simulink model "Thirtybussys_final"  (R2023b)
settings: Solver=VariableStepAuto  StartTime=0.0  StopTime=0.7  RelTol=1e-3
libraries: eePowerMeasurement x60, spsFourierLib x60, spsThreePhaseSeriesRLCBranchLib x41, spsThreePhaseVIMeasurementLib x30, spsThreePhaseSeriesRLCLoadLib x21, spsThreePhaseSourceLib x6, spsThreePhaseTransformerTwoWindingsLib x6, spsThreePhaseFaultLib x2, spspowerguiLib x1
(part 1 of 3)
settings Model: Creator=sariy sh  LastModifiedBy=HP
settings SolverCC: AlgebraicLoopSolver=TrustRegion
settings DataIOCC: ReturnWorkspaceOutputs=off
settings DebuggingCC: UnconnectedInputMsg=warning  UnconnectedOutputMsg=warning  UnconnectedLineMsg=warning  ArithmeticOperatorsInVariantConditions=warning
settings ModelReferenceCC: EnableRefExpFcnMdlSchedulingChecks=on
settings SFSimCC: SimUseLocalCustomCode=off  CustomCodeUndefinedFunction=UseInterfaceOnly
settings RTWCC: RTWUseLocalCustomCode=off
settings CodeAppCC: StateflowObjectComments=on
settings SimscapeCC: SimscapeNormalizeSystem=off

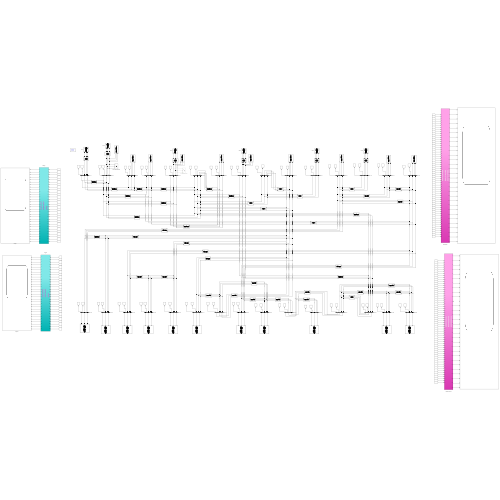
[thumbnail: Simulink's stored preview of the top-level diagram]
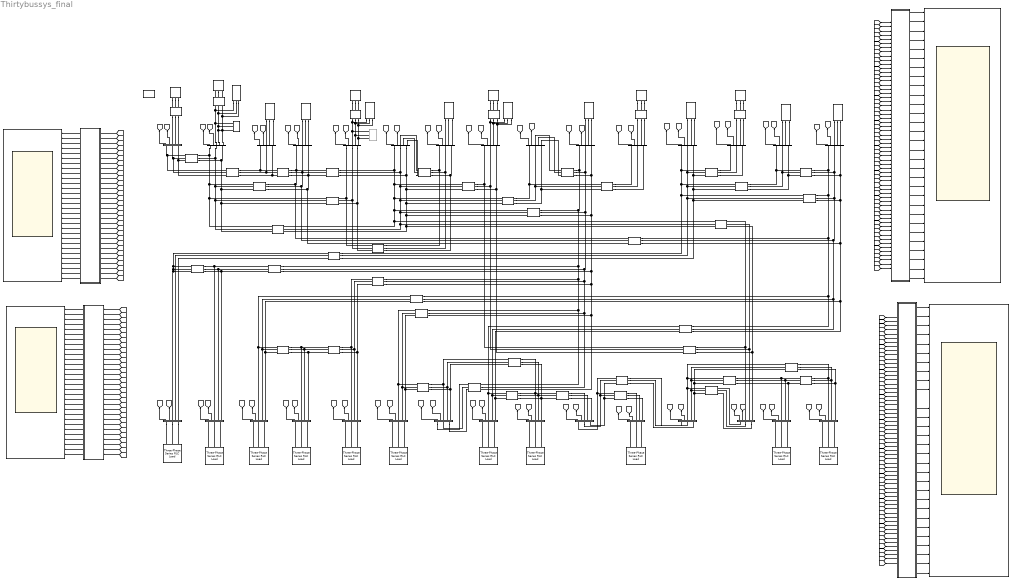
== system Thirtybussys_final ==
  " Reactive Power" : Subsystem
  " Real Power" : Subsystem
  Bus {1..30} (30 alike) : spsThreePhaseVIMeasurementLib/Three-Phase V-I Measurement  VoltageMeasurement=phase-to-ground  SetLabelV=off  LabelV=Vabc  Vpu=off  VpuLL=off  CurrentMeasurement=yes  SetLabelI=off  LabelI=Iabc  Ipu=off  Pbase=100e6  Vbase=500e3  OutputType=Complex  PhasorSimulation=off  PSBequivalent=0
  Current 1 : Subsystem
  Gen1 : spsThreePhaseSourceLib/Three-Phase Source  InternalConnection=Yg  VoltagePhases=off  Voltage=1.06  PhaseAngle=0  Voltage_phases=[25e3 25e3 25e3]/sqrt(3)  PhaseAngles_phases=[0 -120 +120]  Frequency=50  NonIdealSource=on  SpecifyImpedance=on  Resistance=0.8929  Inductance=16.58e-3  ShortCircuitLevel=100e6  BaseVoltage=1  XRratio=1  BusType=swing  Pref=10e3  Qref=0  Prefabc=[10e3, 10e3, 10e3]  Qrefabc=[0, 0, 0]  Qmin=-inf  Qmax=inf
  Gen2 : spsThreePhaseSourceLib/Three-Phase Source  InternalConnection=Yg  VoltagePhases=off  Voltage=1.045  PhaseAngle=0  Voltage_phases=[25e3 25e3 25e3]/sqrt(3)  PhaseAngles_phases=[0 -120 +120]  Frequency=50  NonIdealSource=on  SpecifyImpedance=on  Resistance=0.8929  Inductance=16.58e-3  ShortCircuitLevel=100e6  BaseVoltage=1  XRratio=1  BusType=PQ  Pref=0.4  Qref=0.5  Prefabc=[10e3, 10e3, 10e3]  Qrefabc=[0, 0, 0]  Qmin=-inf  Qmax=inf
  Gen3 : spsThreePhaseSourceLib/Three-Phase Source  InternalConnection=Yg  VoltagePhases=off  Voltage=1.010  PhaseAngle=0  Voltage_phases=[25e3 25e3 25e3]/sqrt(3)  PhaseAngles_phases=[0 -120 +120]  Frequency=50  NonIdealSource=on  SpecifyImpedance=on  Resistance=0.8929  Inductance=16.58e-3  ShortCircuitLevel=100e6  BaseVoltage=1  XRratio=1  BusType=PV  Pref=0.37  Qref=0  Prefabc=[10e3, 10e3, 10e3]  Qrefabc=[0, 0, 0]  Qmin=-0.15  Qmax=0.625
  Gen4 : spsThreePhaseSourceLib/Three-Phase Source  InternalConnection=Yg  VoltagePhases=off  Voltage=1.010  PhaseAngle=0  Voltage_phases=[25e3 25e3 25e3]/sqrt(3)  PhaseAngles_phases=[0 -120 +120]  Frequency=50  NonIdealSource=on  SpecifyImpedance=on  Resistance=0.8929  Inductance=16.58e-3  ShortCircuitLevel=100e6  BaseVoltage=1  XRratio=1  BusType=PV  Pref=0.373  Qref=0  Prefabc=[10e3, 10e3, 10e3]  Qrefabc=[0, 0, 0]  Qmin=-0.15  Qmax=0.50
  Gen5 : spsThreePhaseSourceLib/Three-Phase Source  InternalConnection=Yg  VoltagePhases=off  Voltage=1.082  PhaseAngle=0  Voltage_phases=[25e3 25e3 25e3]/sqrt(3)  PhaseAngles_phases=[0 -120 +120]  Frequency=50  NonIdealSource=on  SpecifyImpedance=on  Resistance=0.8929  Inductance=16.58e-3  ShortCircuitLevel=100e6  BaseVoltage=1  XRratio=1  BusType=PV  Pref=0.162  Qref=0  Prefabc=[10e3, 10e3, 10e3]  Qrefabc=[0, 0, 0]  Qmin=-0.10  Qmax=0.40
  Gen6 : spsThreePhaseSourceLib/Three-Phase Source  InternalConnection=Yg  VoltagePhases=off  Voltage=1.071  PhaseAngle=0  Voltage_phases=[25e3 25e3 25e3]/sqrt(3)  PhaseAngles_phases=[0 -120 +120]  Frequency=50  NonIdealSource=on  SpecifyImpedance=on  Resistance=0.8929  Inductance=16.58e-3  ShortCircuitLevel=100e6  BaseVoltage=1  XRratio=1  BusType=PV  Pref=0.106  Qref=0  Prefabc=[10e3, 10e3, 10e3]  Qrefabc=[0, 0, 0]  Qmin=-0.15  Qmax=0.45
  Reactive Power : Scope  NumInputPorts=30
  Real Power : Scope  NumInputPorts=30
  Scope1 : Scope  NumInputPorts=30
  Scope2 : Scope  NumInputPorts=30
  Three-Phase Series RLC Branch : spsThreePhaseSeriesRLCBranchLib/Three-Phase Series RLC Branch  LConnTagsString=A|B|C  RConnTagsString=A|B|C  BranchType=RLC  Resistance=0.0192  Inductance=0.0575/(2*pi*50)  Capacitance=1/0.0264/(2*pi*50)  Measurements=None
  Three-Phase Series RLC Branch1 : spsThreePhaseSeriesRLCBranchLib/Three-Phase Series RLC Branch  LConnTagsString=A|B|C  RConnTagsString=A|B|C  BranchType=RLC  Resistance=0.0452  Inductance=0.1652/(2*pi*50)  Capacitance=1/0.0204/(2*pi*50)  Measurements=None
  Three-Phase Series RLC Branch10 : spsThreePhaseSeriesRLCBranchLib/Three-Phase Series RLC Branch  LConnTagsString=A|B|C  RConnTagsString=A|B|C  BranchType=L  Resistance=0  Inductance=0.2080/(2*pi*50)  Capacitance=0  Measurements=None
  Three-Phase Series RLC Branch11 : spsThreePhaseSeriesRLCBranchLib/Three-Phase Series RLC Branch  LConnTagsString=A|B|C  RConnTagsString=A|B|C  BranchType=L  Resistance=1  Inductance=0.1100/(2*pi*50)  Capacitance=1e-6  Measurements=None
  Three-Phase Series RLC Branch12 : spsThreePhaseSeriesRLCBranchLib/Three-Phase Series RLC Branch  LConnTagsString=A|B|C  RConnTagsString=A|B|C  BranchType=L  Resistance=1  Inductance=0.5560/(2*pi*50)  Capacitance=1e-6  Measurements=None
  Three-Phase Series RLC Branch13 : spsThreePhaseSeriesRLCBranchLib/Three-Phase Series RLC Branch  LConnTagsString=A|B|C  RConnTagsString=A|B|C  BranchType=L  Resistance=1  Inductance=0.2080/(2*pi*50)  Capacitance=1e-6  Measurements=None
  Three-Phase Series RLC Branch14 : spsThreePhaseSeriesRLCBranchLib/Three-Phase Series RLC Branch  LConnTagsString=A|B|C  RConnTagsString=A|B|C  BranchType=L  Resistance=1  Inductance=0.1400/(2*pi*50)  Capacitance=1e-6  Measurements=None
  Three-Phase Series RLC Branch15 : spsThreePhaseSeriesRLCBranchLib/Three-Phase Series RLC Branch  LConnTagsString=A|B|C  RConnTagsString=A|B|C  BranchType=RL  Resistance=0.1231  Inductance=0.2559/(2*pi*50)  Capacitance=1e-6  Measurements=None
  Three-Phase Series RLC Branch16 : spsThreePhaseSeriesRLCBranchLib/Three-Phase Series RLC Branch  LConnTagsString=A|B|C  RConnTagsString=A|B|C  BranchType=RL  Resistance=0.2210  Inductance=0.1997/(2*pi*50)  Capacitance=1e-6  Measurements=None
  Three-Phase Series RLC Branch17 : spsThreePhaseSeriesRLCBranchLib/Three-Phase Series RLC Branch  LConnTagsString=A|B|C  RConnTagsString=A|B|C  BranchType=L  Resistance=1  Inductance=0.2560/(2*pi*50)  Capacitance=1e-6  Measurements=None
  Three-Phase Series RLC Branch18 : spsThreePhaseSeriesRLCBranchLib/Three-Phase Series RLC Branch  LConnTagsString=A|B|C  RConnTagsString=A|B|C  BranchType=RL  Resistance=0.0945  Inductance=0.1987/(2*pi*50)  Capacitance=1e-6  Measurements=None
  Three-Phase Series RLC Branch19 : spsThreePhaseSeriesRLCBranchLib/Three-Phase Series RLC Branch  LConnTagsString=A|B|C  RConnTagsString=A|B|C  BranchType=RLC  Resistance=0.0524  Inductance=0.1923/(2*pi*50)  Capacitance=1e-6  Measurements=None
  Three-Phase Series RLC Branch2 : spsThreePhaseSeriesRLCBranchLib/Three-Phase Series RLC Branch  LConnTagsString=A|B|C  RConnTagsString=A|B|C  BranchType=RLC  Resistance=0.0132  Inductance=0.0379/(2*pi*50)  Capacitance=1/0.0042/(2*pi*50)  Measurements=None
  Three-Phase Series RLC Branch20 : spsThreePhaseSeriesRLCBranchLib/Three-Phase Series RLC Branch  LConnTagsString=A|B|C  RConnTagsString=A|B|C  BranchType=RL  Resistance=0.0324  Inductance=0.0845/(2*pi*50)  Capacitance=1e-6  Measurements=None
  Three-Phase Series RLC Branch21 : spsThreePhaseSeriesRLCBranchLib/Three-Phase Series RLC Branch  LConnTagsString=A|B|C  RConnTagsString=A|B|C  BranchType=RL  Resistance=0.1063  Inductance=0.2185/(2*pi*50)  Capacitance=1e-6  Measurements=None
  Three-Phase Series RLC Branch22 : spsThreePhaseSeriesRLCBranchLib/Three-Phase Series RLC Branch  LConnTagsString=A|B|C  RConnTagsString=A|B|C  BranchType=RL  Resistance=0.0639  Inductance=0.1292/(2*pi*50)  Capacitance=1e-6  Measurements=None
  Three-Phase Series RLC Branch23 : spsThreePhaseSeriesRLCBranchLib/Three-Phase Series RLC Branch  LConnTagsString=A|B|C  RConnTagsString=A|B|C  BranchType=RL  Resistance=0.0340  Inductance=0.0680/(2*pi*50)  Capacitance=1e-6  Measurements=None
  Three-Phase Series RLC Branch24 : spsThreePhaseSeriesRLCBranchLib/Three-Phase Series RLC Branch  LConnTagsString=A|B|C  RConnTagsString=A|B|C  BranchType=RL  Resistance=0.0936  Inductance=0.2090/(2*pi*50)  Capacitance=1e-6  Measurements=None
  Three-Phase Series RLC Branch25 : spsThreePhaseSeriesRLCBranchLib/Three-Phase Series RLC Branch  LConnTagsString=A|B|C  RConnTagsString=A|B|C  BranchType=RL  Resistance=0.0348  Inductance=0.0749/(2*pi*50)  Capacitance=1e-6  Measurements=None
  Three-Phase Series RLC Branch26 : spsThreePhaseSeriesRLCBranchLib/Three-Phase Series RLC Branch  LConnTagsString=A|B|C  RConnTagsString=A|B|C  BranchType=RL  Resistance=0.0116  Inductance=0.0236/(2*pi*50)  Capacitance=1e-6  Measurements=None
  Three-Phase Series RLC Branch27 : spsThreePhaseSeriesRLCBranchLib/Three-Phase Series RLC Branch  LConnTagsString=A|B|C  RConnTagsString=A|B|C  BranchType=RL  Resistance=0.0727  Inductance=0.1499/(2*pi*50)  Capacitance=1e-6  Measurements=None
  Three-Phase Series RLC Branch28 : spsThreePhaseSeriesRLCBranchLib/Three-Phase Series RLC Branch  LConnTagsString=A|B|C  RConnTagsString=A|B|C  BranchType=RL  Resistance=0.1000  Inductance=0.2020/(2*pi*50)  Capacitance=1e-6  Measurements=None
  Three-Phase Series RLC Branch29 : spsThreePhaseSeriesRLCBranchLib/Three-Phase Series RLC Branch  LConnTagsString=A|B|C  RConnTagsString=A|B|C  BranchType=RL  Resistance=0.1150  Inductance=0.1790/(2*pi*50)  Capacitance=1e-6  Measurements=None
  Three-Phase Series RLC Branch3 : spsThreePhaseSeriesRLCBranchLib/Three-Phase Series RLC Branch  LConnTagsString=A|B|C  RConnTagsString=A|B|C  BranchType=RLC  Resistance=0.0570  Inductance=0.1737/(2*pi*50)  Capacitance=1/0.0184/(2*pi*50)  Measurements=None
  Three-Phase Series RLC Branch30 : spsThreePhaseSeriesRLCBranchLib/Three-Phase Series RLC Branch  LConnTagsString=A|B|C  RConnTagsString=A|B|C  BranchType=RL  Resistance=0.1320  Inductance=0.2700/(2*pi*50)  Capacitance=1e-6  Measurements=None
  Three-Phase Series RLC Branch31 : spsThreePhaseSeriesRLCBranchLib/Three-Phase Series RLC Branch  LConnTagsString=A|B|C  RConnTagsString=A|B|C  BranchType=RL  Resistance=0.1885  Inductance=0.3292/(2*pi*50)  Capacitance=1e-6  Measurements=None
  Three-Phase Series RLC Branch32 : spsThreePhaseSeriesRLCBranchLib/Three-Phase Series RLC Branch  LConnTagsString=A|B|C  RConnTagsString=A|B|C  BranchType=RL  Resistance=0.2544  Inductance=0.3800/(2*pi*50)  Capacitance=1e-6  Measurements=None
  Three-Phase Series RLC Branch33 : spsThreePhaseSeriesRLCBranchLib/Three-Phase Series RLC Branch  LConnTagsString=A|B|C  RConnTagsString=A|B|C  BranchType=RL  Resistance=0.1093  Inductance=0.2087/(2*pi*50)  Capacitance=1e-6  Measurements=None
  Three-Phase Series RLC Branch34 : spsThreePhaseSeriesRLCBranchLib/Three-Phase Series RLC Branch  LConnTagsString=A|B|C  RConnTagsString=A|B|C  BranchType=RL  Resistance=0.2198  Inductance=0.4153/(2*pi*50)  Capacitance=1e-6  Measurements=None
  Three-Phase Series RLC Branch35 : spsThreePhaseSeriesRLCBranchLib/Three-Phase Series RLC Branch  LConnTagsString=A|B|C  RConnTagsString=A|B|C  BranchType=RL  Resistance=0.3202  Inductance=0.6027/(2*pi*50)  Capacitance=1e-6  Measurements=None
  Three-Phase Series RLC Branch36 : spsThreePhaseSeriesRLCBranchLib/Three-Phase Series RLC Branch  LConnTagsString=A|B|C  RConnTagsString=A|B|C  BranchType=L  Resistance=1  Inductance=0.3960/(2*pi*50)  Capacitance=1e-6  Measurements=None
  Three-Phase Series RLC Branch37 : spsThreePhaseSeriesRLCBranchLib/Three-Phase Series RLC Branch  LConnTagsString=A|B|C  RConnTagsString=A|B|C  BranchType=RLC  Resistance=0.0169  Inductance=0.0599/(2*pi*50)  Capacitance=1/0.0065/(2*pi*50)  Measurements=None
  Three-Phase Series RLC Branch38 : spsThreePhaseSeriesRLCBranchLib/Three-Phase Series RLC Branch  LConnTagsString=A|B|C  RConnTagsString=A|B|C  BranchType=RLC  Resistance=0.0636  Inductance=0.2000/(2*pi*50)  Capacitance=1/0.0214/(2*pi*50)  Measurements=None
  Three-Phase Series RLC Branch39 : spsThreePhaseSeriesRLCBranchLib/Three-Phase Series RLC Branch  LConnTagsString=A|B|C  RConnTagsString=A|B|C  BranchType=RL  Resistance=0.0662  Inductance=0.1304/(2*pi*50)  Capacitance=1e-6  Measurements=None
  Three-Phase Series RLC Branch4 : spsThreePhaseSeriesRLCBranchLib/Three-Phase Series RLC Branch  LConnTagsString=A|B|C  RConnTagsString=A|B|C  BranchType=RLC  Resistance=0.0472  Inductance=0.1983/(2*pi*50)  Capacitance=1/0.0209/(2*pi*50)  Measurements=None
  Three-Phase Series RLC Branch40 : spsThreePhaseSeriesRLCBranchLib/Three-Phase Series RLC Branch  LConnTagsString=A|B|C  RConnTagsString=A|B|C  BranchType=RL  Resistance=0.2399  Inductance=0.4533/(2*pi*50)  Capacitance=1e-6  Measurements=None
  Three-Phase Series RLC Branch5 : spsThreePhaseSeriesRLCBranchLib/Three-Phase Series RLC Branch  LConnTagsString=A|B|C  RConnTagsString=A|B|C  BranchType=RLC  Resistance=0.0581  Inductance=0.1763/(2*pi*50)  Capacitance=1/0.0187/(2*pi*50)  Measurements=None
  Three-Phase Series RLC Branch6 : spsThreePhaseSeriesRLCBranchLib/Three-Phase Series RLC Branch  LConnTagsString=A|B|C  RConnTagsString=A|B|C  BranchType=RLC  Resistance=0.0119  Inductance=0.0414/(2*pi*50)  Capacitance=1/0.0045/(2*pi*50)  Measurements=None
  Three-Phase Series RLC Branch7 : spsThreePhaseSeriesRLCBranchLib/Three-Phase Series RLC Branch  LConnTagsString=A|B|C  RConnTagsString=A|B|C  BranchType=RLC  Resistance=0.0267  Inductance=0.0820/(2*pi*50)  Capacitance=1/0.0085/(2*pi*50)  Measurements=None
  Three-Phase Series RLC Branch8 : spsThreePhaseSeriesRLCBranchLib/Three-Phase Series RLC Branch  LConnTagsString=A|B|C  RConnTagsString=A|B|C  BranchType=RLC  Resistance=0.0460  Inductance=0.1160/(2*pi*50)  Capacitance=1/0.0102/(2*pi*50)  Measurements=None
  Three-Phase Series RLC Branch9 : spsThreePhaseSeriesRLCBranchLib/Three-Phase Series RLC Branch  LConnTagsString=A|B|C  RConnTagsString=A|B|C  BranchType=RLC  Resistance=0.0120  Inductance=0.0420/(2*pi*50)  Capacitance=1/0.0045/(2*pi*50)  Measurements=None
  Three-Phase Series RLC Load : spsThreePhaseSeriesRLCLoadLib/Three-Phase Series RLC Load  LConnTagsString=A|B|C  Configuration=Y (grounded)  NominalVoltage=1  Vabc=[1e3 1e3 1e3]  Vabcp=[1e3 1e3 1e3]  NominalFrequency=50  UnbalancedPower=off  ActivePower=0.217  InductivePower=0.127  CapacitivePower=0  Pabc=[10e3 9e3 11e3]  QLabc=[100 90 110]  QCabc=[100 90 110]  Pabcp=[10e3 9e3 11e3]  QLabcp=[100 90 110]  QCabcp=[100 90 110]  Measurements=None  LoadType=constant Z
  Three-Phase Series RLC Load1 : spsThreePhaseSeriesRLCLoadLib/Three-Phase Series RLC Load  LConnTagsString=A|B|C  Configuration=Y (grounded)  NominalVoltage=1  Vabc=[1e3 1e3 1e3]  Vabcp=[1e3 1e3 1e3]  NominalFrequency=50  UnbalancedPower=off  ActivePower=0.024  InductivePower=0.012  CapacitivePower=0  Pabc=[10e3 9e3 11e3]  QLabc=[100 90 110]  QCabc=[100 90 110]  Pabcp=[10e3 9e3 11e3]  QLabcp=[100 90 110]  QCabcp=[100 90 110]  Measurements=None  LoadType=constant Z
  Three-Phase Series RLC Load10 : spsThreePhaseSeriesRLCLoadLib/Three-Phase Series RLC Load  LConnTagsString=A|B|C  Configuration=Y (grounded)  NominalVoltage=1  Vabc=[1e3 1e3 1e3]  Vabcp=[1e3 1e3 1e3]  NominalFrequency=50  UnbalancedPower=off  ActivePower=0.062  InductivePower=0.016  CapacitivePower=0  Pabc=[10e3 9e3 11e3]  QLabc=[100 90 110]  QCabc=[100 90 110]  Pabcp=[10e3 9e3 11e3]  QLabcp=[100 90 110]  QCabcp=[100 90 110]  Measurements=None  LoadType=constant Z
  Three-Phase Series RLC Load11 : spsThreePhaseSeriesRLCLoadLib/Three-Phase Series RLC Load  LConnTagsString=A|B|C  Configuration=Y (grounded)  NominalVoltage=1  Vabc=[1e3 1e3 1e3]  Vabcp=[1e3 1e3 1e3]  NominalFrequency=50  UnbalancedPower=off  ActivePower=0.082  InductivePower=0.025  CapacitivePower=0  Pabc=[10e3 9e3 11e3]  QLabc=[100 90 110]  QCabc=[100 90 110]  Pabcp=[10e3 9e3 11e3]  QLabcp=[100 90 110]  QCabcp=[100 90 110]  Measurements=None  LoadType=constant Z
  Three-Phase Series RLC Load12 : spsThreePhaseSeriesRLCLoadLib/Three-Phase Series RLC Load  LConnTagsString=A|B|C  Configuration=Y (grounded)  NominalVoltage=1  Vabc=[1e3 1e3 1e3]  Vabcp=[1e3 1e3 1e3]  NominalFrequency=50  UnbalancedPower=off  ActivePower=0.3  InductivePower=0.3  CapacitivePower=0  Pabc=[10e3 9e3 11e3]  QLabc=[100 90 110]  QCabc=[100 90 110]  Pabcp=[10e3 9e3 11e3]  QLabcp=[100 90 110]  QCabcp=[100 90 110]  Measurements=None  LoadType=constant Z
  Three-Phase Series RLC Load13 : spsThreePhaseSeriesRLCLoadLib/Three-Phase Series RLC Load  LConnTagsString=A|B|C  Configuration=Y (grounded)  NominalVoltage=1  Vabc=[1e3 1e3 1e3]  Vabcp=[1e3 1e3 1e3]  NominalFrequency=50  UnbalancedPower=off  ActivePower=0.032  InductivePower=0.009  CapacitivePower=0  Pabc=[10e3 9e3 11e3]  QLabc=[100 90 110]  QCabc=[100 90 110]  Pabcp=[10e3 9e3 11e3]  QLabcp=[100 90 110]  QCabcp=[100 90 110]  Measurements=None  LoadType=constant Z
  Three-Phase Series RLC Load14 : spsThreePhaseSeriesRLCLoadLib/Three-Phase Series RLC Load  LConnTagsString=A|B|C  Configuration=Y (grounded)  NominalVoltage=1  Vabc=[1e3 1e3 1e3]  Vabcp=[1e3 1e3 1e3]  NominalFrequency=50  UnbalancedPower=off  ActivePower=0.095  InductivePower=0.034  CapacitivePower=0  Pabc=[10e3 9e3 11e3]  QLabc=[100 90 110]  QCabc=[100 90 110]  Pabcp=[10e3 9e3 11e3]  QLabcp=[100 90 110]  QCabcp=[100 90 110]  Measurements=None  LoadType=constant Z
  Three-Phase Series RLC Load15 : spsThreePhaseSeriesRLCLoadLib/Three-Phase Series RLC Load  LConnTagsString=A|B|C  Configuration=Y (grounded)  NominalVoltage=1  Vabc=[1e3 1e3 1e3]  Vabcp=[1e3 1e3 1e3]  NominalFrequency=50  UnbalancedPower=off  ActivePower=0.022  InductivePower=0.007  CapacitivePower=0  Pabc=[10e3 9e3 11e3]  QLabc=[100 90 110]  QCabc=[100 90 110]  Pabcp=[10e3 9e3 11e3]  QLabcp=[100 90 110]  QCabcp=[100 90 110]  Measurements=None  LoadType=constant Z
  Three-Phase Series RLC Load16 : spsThreePhaseSeriesRLCLoadLib/Three-Phase Series RLC Load  LConnTagsString=A|B|C  Configuration=Y (grounded)  NominalVoltage=1  Vabc=[1e3 1e3 1e3]  Vabcp=[1e3 1e3 1e3]  NominalFrequency=50  UnbalancedPower=off  ActivePower=0.175  InductivePower=0.112  CapacitivePower=0  Pabc=[10e3 9e3 11e3]  QLabc=[100 90 110]  QCabc=[100 90 110]  Pabcp=[10e3 9e3 11e3]  QLabcp=[100 90 110]  QCabcp=[100 90 110]  Measurements=None  LoadType=constant Z
  Three-Phase Series RLC Load17 : spsThreePhaseSeriesRLCLoadLib/Three-Phase Series RLC Load  LConnTagsString=A|B|C  Configuration=Y (grounded)  NominalVoltage=1  Vabc=[1e3 1e3 1e3]  Vabcp=[1e3 1e3 1e3]  NominalFrequency=50  UnbalancedPower=off  ActivePower=0.032  InductivePower=0.016  CapacitivePower=0  Pabc=[10e3 9e3 11e3]  QLabc=[100 90 110]  QCabc=[100 90 110]  Pabcp=[10e3 9e3 11e3]  QLabcp=[100 90 110]  QCabcp=[100 90 110]  Measurements=None  LoadType=constant Z
  Three-Phase Series RLC Load18 : spsThreePhaseSeriesRLCLoadLib/Three-Phase Series RLC Load  LConnTagsString=A|B|C  Configuration=Y (grounded)  NominalVoltage=1  Vabc=[1e3 1e3 1e3]  Vabcp=[1e3 1e3 1e3]  NominalFrequency=50  UnbalancedPower=off  ActivePower=0.087  InductivePower=0.067  CapacitivePower=0  Pabc=[10e3 9e3 11e3]  QLabc=[100 90 110]  QCabc=[100 90 110]  Pabcp=[10e3 9e3 11e3]  QLabcp=[100 90 110]  QCabcp=[100 90 110]  Measurements=None  LoadType=constant Z
  Three-Phase Series RLC Load19 : spsThreePhaseSeriesRLCLoadLib/Three-Phase Series RLC Load  LConnTagsString=A|B|C  Configuration=Y (grounded)  NominalVoltage=1  Vabc=[1e3 1e3 1e3]  Vabcp=[1e3 1e3 1e3]  NominalFrequency=50  UnbalancedPower=off  ActivePower=0.035  InductivePower=0.023  CapacitivePower=0  Pabc=[10e3 9e3 11e3]  QLabc=[100 90 110]  QCabc=[100 90 110]  Pabcp=[10e3 9e3 11e3]  QLabcp=[100 90 110]  QCabcp=[100 90 110]  Measurements=None  LoadType=constant Z
  Three-Phase Series RLC Load2 : spsThreePhaseSeriesRLCLoadLib/Three-Phase Series RLC Load  LConnTagsString=A|B|C  Configuration=Y (grounded)  NominalVoltage=1  Vabc=[1e3 1e3 1e3]  Vabcp=[1e3 1e3 1e3]  NominalFrequency=50  UnbalancedPower=off  ActivePower=0.076  InductivePower=0.016  CapacitivePower=0  Pabc=[10e3 9e3 11e3]  QLabc=[100 90 110]  QCabc=[100 90 110]  Pabcp=[10e3 9e3 11e3]  QLabcp=[100 90 110]  QCabcp=[100 90 110]  Measurements=None  LoadType=constant Z
  Three-Phase Series RLC Load21 : spsThreePhaseSeriesRLCLoadLib/Three-Phase Series RLC Load  LConnTagsString=A|B|C  Configuration=Y (grounded)  NominalVoltage=1  Vabc=[1e3 1e3 1e3]  Vabcp=[1e3 1e3 1e3]  NominalFrequency=50  UnbalancedPower=off  ActivePower=0.024  InductivePower=0.009  CapacitivePower=0  Pabc=[10e3 9e3 11e3]  QLabc=[100 90 110]  QCabc=[100 90 110]  Pabcp=[10e3 9e3 11e3]  QLabcp=[100 90 110]  QCabcp=[100 90 110]  Measurements=None  LoadType=constant Z
  Three-Phase Series RLC Load22 : spsThreePhaseSeriesRLCLoadLib/Three-Phase Series RLC Load  LConnTagsString=A|B|C  Configuration=Y (grounded)  NominalVoltage=1  Vabc=[1e3 1e3 1e3]  Vabcp=[1e3 1e3 1e3]  NominalFrequency=50  UnbalancedPower=off  ActivePower=0.106  InductivePower=0.019  CapacitivePower=0  Pabc=[10e3 9e3 11e3]  QLabc=[100 90 110]  QCabc=[100 90 110]  Pabcp=[10e3 9e3 11e3]  QLabcp=[100 90 110]  QCabcp=[100 90 110]  Measurements=None  LoadType=constant Z
  Three-Phase Series RLC Load3 : spsThreePhaseSeriesRLCLoadLib/Three-Phase Series RLC Load  LConnTagsString=A|B|C  Configuration=Y (grounded)  NominalVoltage=1  Vabc=[1e3 1e3 1e3]  Vabcp=[1e3 1e3 1e3]  NominalFrequency=50  UnbalancedPower=off  ActivePower=0.942  InductivePower=0.19  CapacitivePower=0  Pabc=[10e3 9e3 11e3]  QLabc=[100 90 110]  QCabc=[100 90 110]  Pabcp=[10e3 9e3 11e3]  QLabcp=[100 90 110]  QCabcp=[100 90 110]  Measurements=None  LoadType=constant Z
  Three-Phase Series RLC Load4 : spsThreePhaseSeriesRLCLoadLib/Three-Phase Series RLC Load  LConnTagsString=A|B|C  Configuration=Y (grounded)  NominalVoltage=1  Vabc=[1e3 1e3 1e3]  Vabcp=[1e3 1e3 1e3]  NominalFrequency=50  UnbalancedPower=off  ActivePower=0.09  InductivePower=0.058  CapacitivePower=0  Pabc=[10e3 9e3 11e3]  QLabc=[100 90 110]  QCabc=[100 90 110]  Pabcp=[10e3 9e3 11e3]  QLabcp=[100 90 110]  QCabcp=[100 90 110]  Measurements=None  LoadType=constant Z
  Three-Phase Series RLC Load5 : spsThreePhaseSeriesRLCLoadLib/Three-Phase Series RLC Load  LConnTagsString=A|B|C  Configuration=Y (grounded)  NominalVoltage=1  Vabc=[1e3 1e3 1e3]  Vabcp=[1e3 1e3 1e3]  NominalFrequency=50  UnbalancedPower=off  ActivePower=0.228  InductivePower=0.109  CapacitivePower=0  Pabc=[10e3 9e3 11e3]  QLabc=[100 90 110]  QCabc=[100 90 110]  Pabcp=[10e3 9e3 11e3]  QLabcp=[100 90 110]  QCabcp=[100 90 110]  Measurements=None  LoadType=constant Z
  Three-Phase Series RLC Load7 : spsThreePhaseSeriesRLCLoadLib/Three-Phase Series RLC Load  LConnTagsString=A|B|C  Configuration=Y (grounded)  NominalVoltage=1  Vabc=[1e3 1e3 1e3]  Vabcp=[1e3 1e3 1e3]  NominalFrequency=50  UnbalancedPower=off  ActivePower=0.058  InductivePower=0.02  CapacitivePower=0  Pabc=[10e3 9e3 11e3]  QLabc=[100 90 110]  QCabc=[100 90 110]  Pabcp=[10e3 9e3 11e3]  QLabcp=[100 90 110]  QCabcp=[100 90 110]  Measurements=None  LoadType=constant Z
  Three-Phase Series RLC Load8 : spsThreePhaseSeriesRLCLoadLib/Three-Phase Series RLC Load  LConnTagsString=A|B|C  Configuration=Y (grounded)  NominalVoltage=1  Vabc=[1e3 1e3 1e3]  Vabcp=[1e3 1e3 1e3]  NominalFrequency=50  UnbalancedPower=off  ActivePower=0.09  InductivePower=0.058  CapacitivePower=0  Pabc=[10e3 9e3 11e3]  QLabc=[100 90 110]  QCabc=[100 90 110]  Pabcp=[10e3 9e3 11e3]  QLabcp=[100 90 110]  QCabcp=[100 90 110]  Measurements=None  LoadType=constant Z
  Three-Phase Series RLC Load9 : spsThreePhaseSeriesRLCLoadLib/Three-Phase Series RLC Load  LConnTagsString=A|B|C  Configuration=Y (grounded)  NominalVoltage=1  Vabc=[1e3 1e3 1e3]  Vabcp=[1e3 1e3 1e3]  NominalFrequency=50  UnbalancedPower=off  ActivePower=0.112  InductivePower=0.075  CapacitivePower=0  Pabc=[10e3 9e3 11e3]  QLabc=[100 90 110]  QCabc=[100 90 110]  Pabcp=[10e3 9e3 11e3]  QLabcp=[100 90 110]  QCabcp=[100 90 110]  Measurements=None  LoadType=constant Z
  Three-Phase Transformer (Two Windings) : spsThreePhaseTransformerTwoWindingsLib/Three-Phase Transformer (Two Windings)  Winding1Connection=Yg  Winding2Connection=Yg  CoreType=Three single-phase transformers  SetSaturation=off  Hysteresis=off  DataFile='hysteresis'  SetInitialFlux=off  Measurements=None  UNITS=pu  NominalPower=[ 1 , 50 ]  Winding1=[1.06 , 0.002 , 0.08 ]  Winding2=[ 1.06 , 0.002 , 0.08 ]  Rm=500  Lm=500  L0=0.5  Saturation=[ 0,0 ; 0.0024,1.2 ; 1.0,1.52 ]  InitialFluxes=[ 0.8 , -0.8 , 0.7 ]  BreakLoop=off  DiscreteSolver=Trapezoidal iterative  DataType=off  TransfoNumber=1
  Three-Phase Transformer (Two Windings)1 : spsThreePhaseTransformerTwoWindingsLib/Three-Phase Transformer (Two Windings)  Winding1Connection=Yg  Winding2Connection=Yg  CoreType=Three single-phase transformers  SetSaturation=off  Hysteresis=off  DataFile='hysteresis'  SetInitialFlux=off  Measurements=None  UNITS=pu  NominalPower=[1 , 50 ]  Winding1=[ 1.045 , 0.002 , 0.08 ]  Winding2=[ 1.045 , 0.002 , 0.08 ]  Rm=500  Lm=500  L0=0.5  Saturation=[ 0,0 ; 0.0024,1.2 ; 1.0,1.52 ]  InitialFluxes=[ 0.8 , -0.8 , 0.7 ]  BreakLoop=off  DiscreteSolver=Trapezoidal iterative  DataType=off  TransfoNumber=1
  Three-Phase Transformer (Two Windings)2 : spsThreePhaseTransformerTwoWindingsLib/Three-Phase Transformer (Two Windings)  Winding1Connection=Yg  Winding2Connection=Yg  CoreType=Three single-phase transformers  SetSaturation=off  Hysteresis=off  DataFile='hysteresis'  SetInitialFlux=off  Measurements=None  UNITS=pu  NominalPower=[ 1 , 50 ]  Winding1=[ 1.010 , 0.002 , 0.08 ]  Winding2=[ 1.010 , 0.002 , 0.08 ]  Rm=500  Lm=500  L0=0.5  Saturation=[ 0,0 ; 0.0024,1.2 ; 1.0,1.52 ]  InitialFluxes=[ 0.8 , -0.8 , 0.7 ]  BreakLoop=off  DiscreteSolver=Trapezoidal iterative  DataType=off  TransfoNumber=1
  Three-Phase Transformer (Two Windings)3 : spsThreePhaseTransformerTwoWindingsLib/Three-Phase Transformer (Two Windings)  Winding1Connection=Yg  Winding2Connection=Yg  CoreType=Three single-phase transformers  SetSaturation=off  Hysteresis=off  DataFile='hysteresis'  SetInitialFlux=off  Measurements=None  UNITS=pu  NominalPower=[ 250e6 , 60 ]  Winding1=[ 735e3 , 0.002 , 0.08 ]  Winding2=[ 315e3 , 0.002 , 0.08 ]  Rm=500  Lm=500  L0=0.5  Saturation=[ 0,0 ; 0.0024,1.2 ; 1.0,1.52 ]  InitialFluxes=[ 0.8 , -0.8 , 0.7 ]  BreakLoop=off  DiscreteSolver=Trapezoidal iterative  DataType=off  TransfoNumber=1
  Three-Phase Transformer (Two Windings)4 : spsThreePhaseTransformerTwoWindingsLib/Three-Phase Transformer (Two Windings)  Winding1Connection=Yg  Winding2Connection=Yg  CoreType=Three single-phase transformers  SetSaturation=off  Hysteresis=off  DataFile='hysteresis'  SetInitialFlux=off  Measurements=None  UNITS=pu  NominalPower=[ 1 , 50 ]  Winding1=[ 1.082 , 0.002 , 0.08 ]  Winding2=[ 1.082 , 0.002 , 0.08 ]  Rm=500  Lm=500  L0=0.5  Saturation=[ 0,0 ; 0.0024,1.2 ; 1.0,1.52 ]  InitialFluxes=[ 0.8 , -0.8 , 0.7 ]  BreakLoop=off  DiscreteSolver=Trapezoidal iterative  DataType=off  TransfoNumber=1
  Three-Phase Transformer (Two Windings)5 : spsThreePhaseTransformerTwoWindingsLib/Three-Phase Transformer (Two Windings)  Winding1Connection=Yg  Winding2Connection=Yg  CoreType=Three single-phase transformers  SetSaturation=off  Hysteresis=off  DataFile='hysteresis'  SetInitialFlux=off  Measurements=None  UNITS=pu  NominalPower=[ 1 , 50 ]  Winding1=[ 1.071 , 0.002 , 0.08 ]  Winding2=[ 1.071 , 0.002 , 0.08 ]  Rm=500  Lm=500  L0=0.5  Saturation=[ 0,0 ; 0.0024,1.2 ; 1.0,1.52 ]  InitialFluxes=[ 0.8 , -0.8 , 0.7 ]  BreakLoop=off  DiscreteSolver=Trapezoidal iterative  DataType=off  TransfoNumber=1
  Three-Phase Fault1 : spsThreePhaseFaultLib/Three-Phase Fault  Commented=on  InitialStates=0  FaultA=on  FaultB=on  FaultC=on  GroundFault=on  SwitchTimes="[0.4  0.5]"  External=off  SwitchStatus=NaN  FaultResistance=0.001  GroundResistance=0.01  SnubberResistance=1e6  SnubberCapacitance=inf  Measurements=None
  Three-Phase Fault2 : spsThreePhaseFaultLib/Three-Phase Fault  InitialStates=0  FaultA=on  FaultB=on  FaultC=on  GroundFault=on  SwitchTimes="[0.4  0.5]"  External=off  SwitchStatus=NaN  FaultResistance=0.01  GroundResistance=0.01  SnubberResistance=1e6  SnubberCapacitance=inf  Measurements=None
  "Voltage " : Subsystem
  powergui : spspowerguiLib/powergui  Priority=1  SimulationMode=Discrete  SampleTime=50e-6  frequency=60  Iterations=50  frequencyindice=50  Pbase=100e6  ErrMax=1e-4  UnitsV=kV  UnitsW=MW  buscounter=0  FunctionMessages=off  echomessages=off  EnableUseOfTLC=off  CurrentSourceSwitches=off  DisableSnubberDevices=off  DisableRonSwitches=off  DisableVfSwitches=off  DisplayEquations=off  AutomaticDiscreteSolvers=off  SolverType=Tustin/Backward Euler (TBE)  Interpol=off  ExternalGateDelay=off  methode=off  Ts=100  x0status=blocks  SPID=off  SwTol=0  HookPort=off  NonlinearTolerance=1e-4  nMaxIteration=100  ContinueOnMaxIteration=off  RestoreLinks=warning  ResistiveCurrentMeasurement=off  Frange=[0:2:500]  Ylog=off  Xlog=on  ShowGrid=off  save=off  variable=ZData  structure=0  ZoomFFT=off  StartTime=0.0  cycles=1  DisplayStyle=1  fundamental=60  FreqAxis=off  MaxFrequency=1000  frequencyindicesteady=1  RmsSteady=1  display=off
  wires:
  Bus 4/1 -> [V4]
  Bus 4/2 -> [I4]
  Bus 5/1 -> [V5]
  Bus 5/2 -> [I5]
  Bus 6/1 -> [V6]
  Bus 6/2 -> [I6]
  Bus 12/1 -> [V12]
  Bus 12/2 -> [I12]
  Bus 13/1 -> [V13]
  Bus 13/2 -> [I13]
  Bus 14/1 -> [V14]
  Bus 14/2 -> [I14]
  Bus 15/1 -> [V15]
  Bus 15/2 -> [I15]
  Bus 16/1 -> [V16]
  Bus 16/2 -> [I16]
  Bus 17/1 -> [V17]
  Bus 17/2 -> [I17]
  Bus 18/1 -> [V18]
  Bus 18/2 -> [I18]
  Bus 19/1 -> [V19]
  Bus 19/2 -> [I19]
  Bus 20/1 -> [V20]
  Bus 20/2 -> [I20]
  Bus 21/1 -> [V21]
  Bus 21/2 -> [I21]
  Bus 22/1 -> [V22]
  Bus 22/2 -> [I22]
  Bus 23/1 -> [V23]
  Bus 23/2 -> [I23]
  Bus 24/1 -> [V24]
  Bus 24/2 -> [I24]
  Bus 25/1 -> [V25]
  Bus 25/2 -> [I25]
  Bus 26/1 -> [V26]
  Bus 26/2 -> [I26]
  Bus 27/1 -> [V27]
  Bus 27/2 -> [I27]
  Bus 28/1 -> [V28]
  Bus 28/2 -> [I28]
  Bus 29/1 -> [V29]
  Bus 29/2 -> [I29]
  Bus 30/1 -> [V30]
  Bus 30/2 -> [I30]
  Bus 2/2 -> [I2]
  Bus 3/2 -> [I3]
  Bus 3/1 -> [V3]
  Bus 1/2 -> [I1]
  Bus 1/1 -> [V1]
  Bus 2/1 -> [V2]
  Bus 7/1 -> [V7]
  Bus 8/1 -> [V8]
  Bus 9/1 -> [V9]
  Bus 10/1 -> [V10]
  Bus 7/2 -> [I7]
  Bus 8/2 -> [I8]
  Bus 9/2 -> [I9]
  Bus 10/2 -> [I10]
  Bus 11/1 -> [V11]
  Bus 11/2 -> [I11]
  [I7] -> Current 1/7(In7)
  [I26] -> Current 1/26(In26)
  [V18] -> "Voltage "/18(In18)
  [V14] -> "Voltage "/14(In14)
  "Voltage "/14(Out14) -> Scope1/14
  "Voltage "/24(Out24) -> Scope1/24
  "Voltage "/10(Out10) -> Scope1/10
  "Voltage "/17(Out17) -> Scope1/17
  "Voltage "/29(Out29) -> Scope1/29
  "Voltage "/16(Out16) -> Scope1/16
  [V11] -> "Voltage "/11(In11)
  "Voltage "/5(Out5) -> Scope1/5
  "Voltage "/20(Out20) -> Scope1/20
  [V3] -> "Voltage "/3(In3)
  [V10] -> "Voltage "/10(In10)
  "Voltage "/21(Out21) -> Scope1/21
  "Voltage "/26(Out26) -> Scope1/26
  [V21] -> "Voltage "/21(In21)
  [V9] -> "Voltage "/9(In9)
  "Voltage "/9(Out9) -> Scope1/9
  "Voltage "/7(Out7) -> Scope1/7
  "Voltage "/23(Out23) -> Scope1/23
  "Voltage "/30(Out30) -> Scope1/30
  "Voltage "/6(Out6) -> Scope1/6
  "Voltage "/22(Out22) -> Scope1/22
  "Voltage "/28(Out28) -> Scope1/28
  [V19] -> "Voltage "/19(In19)
  "Voltage "/8(Out8) -> Scope1/8
  [V1] -> "Voltage "/1(In1)
  [V6] -> "Voltage "/6(In6)
  [V26] -> "Voltage "/26(In26)
  [V20] -> "Voltage "/20(In20)
  [V27] -> "Voltage "/27(In27)
  "Voltage "/15(Out15) -> Scope1/15
  [V25] -> "Voltage "/25(In25)
  [V28] -> "Voltage "/28(In28)
  "Voltage "/13(Out13) -> Scope1/13
  [V4] -> "Voltage "/4(In4)
  [V5] -> "Voltage "/5(In5)
  [V29] -> "Voltage "/29(In29)
  [V7] -> "Voltage "/7(In7)
  [V8] -> "Voltage "/8(In8)
  [V16] -> "Voltage "/16(In16)
  "Voltage "/19(Out19) -> Scope1/19
  [V30] -> "Voltage "/30(In30)
  "Voltage "/12(Out12) -> Scope1/12
  [V13] -> "Voltage "/13(In13)
  "Voltage "/11(Out11) -> Scope1/11
  "Voltage "/3(Out3) -> Scope1/3
  [V2] -> "Voltage "/2(In2)
  "Voltage "/27(Out27) -> Scope1/27
  "Voltage "/2(Out2) -> Scope1/2
  [V15] -> "Voltage "/15(In15)
  "Voltage "/1(Out1) -> Scope1/1
  "Voltage "/18(Out18) -> Scope1/18
  [V24] -> "Voltage "/24(In24)
  [V22] -> "Voltage "/22(In22)
  [I9] -> Current 1/9(In9)
  [I8] -> Current 1/8(In8)
  [I13] -> Current 1/13(In13)
  [I3] -> Current 1/3(In3)
  [I14] -> Current 1/14(In14)
  [I4] -> Current 1/4(In4)
  [I10] -> Current 1/10(In10)
  Current 1/22(Out22) -> Scope2/22
  Current 1/7(Out7) -> Scope2/7
  Current 1/9(Out9) -> Scope2/9
  Current 1/14(Out14) -> Scope2/14
  Current 1/18(Out18) -> Scope2/18
  [I29] -> Current 1/29(In29)
  "Voltage "/4(Out4) -> Scope1/4
  Current 1/25(Out25) -> Scope2/25
  Current 1/4(Out4) -> Scope2/4
  Current 1/29(Out29) -> Scope2/29
  "Voltage "/25(Out25) -> Scope1/25
  [I15] -> Current 1/15(In15)
  Current 1/21(Out21) -> Scope2/21
  [I6] -> Current 1/6(In6)
  [I30] -> Current 1/30(In30)
  Current 1/15(Out15) -> Scope2/15
  Current 1/19(Out19) -> Scope2/19
  Current 1/13(Out13) -> Scope2/13
  [V12] -> "Voltage "/12(In12)
  Current 1/20(Out20) -> Scope2/20
  Current 1/30(Out30) -> Scope2/30
  [I18] -> Current 1/18(In18)
  Current 1/3(Out3) -> Scope2/3
  Current 1/6(Out6) -> Scope2/6
  Current 1/26(Out26) -> Scope2/26
  Current 1/23(Out23) -> Scope2/23
  Current 1/16(Out16) -> Scope2/16
  Current 1/24(Out24) -> Scope2/24
  Current 1/10(Out10) -> Scope2/10
  [I5] -> Current 1/5(In5)
  [I28] -> Current 1/28(In28)
  Current 1/5(Out5) -> Scope2/5
  Current 1/28(Out28) -> Scope2/28
  Current 1/1(Out1) -> Scope2/1
  Current 1/11(Out11) -> Scope2/11
  [I25] -> Current 1/25(In25)
  [I17] -> Current 1/17(In17)
  [I27] -> Current 1/27(In27)
  Current 1/2(Out2) -> Scope2/2
  [I16] -> Current 1/16(In16)
  [I22] -> Current 1/22(In22)
  [I2] -> Current 1/2(In2)
  Current 1/27(Out27) -> Scope2/27
  Current 1/17(Out17) -> Scope2/17
  Current 1/8(Out8) -> Scope2/8
  [I21] -> Current 1/21(In21)
  [V17] -> "Voltage "/17(In17)
  [I19] -> Current 1/19(In19)
  [I11] -> Current 1/11(In11)
  [I24] -> Current 1/24(In24)
  [I12] -> Current 1/12(In12)
  [I20] -> Current 1/20(In20)
  [V23] -> "Voltage "/23(In23)
  Current 1/12(Out12) -> Scope2/12
  [I1] -> Current 1/1(In1)
  [I23] -> Current 1/23(In23)
  " Real Power"/21(Out21) -> Real Power/21
  [I11] -> " Real Power"/22(In22)
  [V11] -> " Real Power"/21(In21)
  [V22] -> " Reactive Power"/43(In43)
  [V11] -> " Reactive Power"/21(In21)
  [V21] -> " Reactive Power"/41(In41)
  [I21] -> " Reactive Power"/42(In42)
  [V3] -> " Reactive Power"/5(In5)
  " Reactive Power"/10(Out10) -> Reactive Power/10
  [I10] -> " Reactive Power"/20(In20)
  [V9] -> " Reactive Power"/17(In17)
  [V10] -> " Reactive Power"/19(In19)
  [I9] -> " Reactive Power"/18(In18)
  [I7] -> " Reactive Power"/14(In14)
  [I8] -> " Reactive Power"/16(In16)
  [V7] -> " Reactive Power"/13(In13)
  " Reactive Power"/6(Out6) -> Reactive Power/6
  " Reactive Power"/4(Out4) -> Reactive Power/4
  [V6] -> " Reactive Power"/11(In11)
  [I6] -> " Reactive Power"/12(In12)
  [V4] -> " Reactive Power"/7(In7)
  [V5] -> " Reactive Power"/9(In9)
  " Reactive Power"/7(Out7) -> Reactive Power/7
  [I3] -> " Reactive Power"/6(In6)
  " Reactive Power"/3(Out3) -> Reactive Power/3
  [V22] -> " Real Power"/43(In43)
  " Reactive Power"/21(Out21) -> Reactive Power/21
  " Reactive Power"/1(Out1) -> Reactive Power/1
  " Real Power"/1(Out1) -> Real Power/1
  [I1] -> " Real Power"/2(In2)
  [I1] -> " Reactive Power"/2(In2)
  [V10] -> " Real Power"/19(In19)
  [I9] -> " Real Power"/18(In18)
  [V4] -> " Real Power"/7(In7)
  [I4] -> " Real Power"/8(In8)
  " Real Power"/27(Out27) -> Real Power/27
  " Real Power"/29(Out29) -> Real Power/29
  " Real Power"/30(Out30) -> Real Power/30
  " Real Power"/28(Out28) -> Real Power/28
  " Real Power"/24(Out24) -> Real Power/24
  " Real Power"/25(Out25) -> Real Power/25
  " Real Power"/26(Out26) -> Real Power/26
  " Real Power"/23(Out23) -> Real Power/23
  [I20] -> " Real Power"/40(In40)
  [V5] -> " Real Power"/9(In9)
  " Real Power"/6(Out6) -> Real Power/6
  [V6] -> " Real Power"/11(In11)
  [I6] -> " Real Power"/12(In12)
  [I10] -> " Real Power"/20(In20)
  " Reactive Power"/8(Out8) -> Reactive Power/8
  [I2] -> " Real Power"/4(In4)
  " Real Power"/15(Out15) -> Real Power/15
  " Real Power"/17(Out17) -> Real Power/17
  " Real Power"/14(Out14) -> Real Power/14
  " Real Power"/13(Out13) -> Real Power/13
  [V3] -> " Real Power"/5(In5)
  [V9] -> " Real Power"/17(In17)
  " Real Power"/5(Out5) -> Real Power/5
  [I3] -> " Real Power"/6(In6)
  [I13] -> " Real Power"/26(In26)
  [V14] -> " Real Power"/27(In27)
  [I14] -> " Real Power"/28(In28)
  [I12] -> " Real Power"/24(In24)
  [V15] -> " Real Power"/29(In29)
  [V13] -> " Real Power"/25(In25)
  [I15] -> " Real Power"/30(In30)
  " Real Power"/2(Out2) -> Real Power/2
  [V2] -> " Real Power"/3(In3)
  [V21] -> " Real Power"/41(In41)
  [V12] -> " Real Power"/23(In23)
  " Real Power"/11(Out11) -> Real Power/11
  " Real Power"/12(Out12) -> Real Power/12
  [I21] -> " Real Power"/42(In42)
  [I22] -> " Reactive Power"/44(In44)
  " Reactive Power"/20(Out20) -> Reactive Power/20
  " Reactive Power"/17(Out17) -> Reactive Power/17
  " Reactive Power"/19(Out19) -> Reactive Power/19
  " Reactive Power"/5(Out5) -> Reactive Power/5
  " Reactive Power"/14(Out14) -> Reactive Power/14
  " Reactive Power"/12(Out12) -> Reactive Power/12
  " Reactive Power"/18(Out18) -> Reactive Power/18
  " Reactive Power"/15(Out15) -> Reactive Power/15
  [V20] -> " Reactive Power"/39(In39)
  [V18] -> " Reactive Power"/35(In35)
  [I19] -> " Reactive Power"/38(In38)
  [I18] -> " Reactive Power"/36(In36)
  [V17] -> " Reactive Power"/33(In33)
  [I17] -> " Reactive Power"/34(In34)
  [I16] -> " Reactive Power"/32(In32)
  [V16] -> " Reactive Power"/31(In31)
  [I11] -> " Reactive Power"/22(In22)
  [V13] -> " Reactive Power"/25(In25)
  [I14] -> " Reactive Power"/28(In28)
  [V15] -> " Reactive Power"/29(In29)
  [V14] -> " Reactive Power"/27(In27)
  [I12] -> " Reactive Power"/24(In24)
  [V1] -> " Real Power"/1(In1)
  [V12] -> " Reactive Power"/23(In23)
  [V2] -> " Reactive Power"/3(In3)
  [V23] -> " Reactive Power"/45(In45)
  [I2] -> " Reactive Power"/4(In4)
  " Reactive Power"/30(Out30) -> Reactive Power/30
  " Real Power"/3(Out3) -> Real Power/3
  " Reactive Power"/27(Out27) -> Reactive Power/27
  [V30] -> " Reactive Power"/59(In59)
  [V26] -> " Reactive Power"/51(In51)
  [V24] -> " Reactive Power"/47(In47)
  " Real Power"/16(Out16) -> Real Power/16
  [I18] -> " Real Power"/36(In36)
  [V18] -> " Real Power"/35(In35)
  [I19] -> " Real Power"/38(In38)
  [V17] -> " Real Power"/33(In33)
  [I27] -> " Reactive Power"/54(In54)
  [I30] -> " Real Power"/60(In60)
  [I29] -> " Real Power"/58(In58)
  [I5] -> " Reactive Power"/10(In10)
  [I27] -> " Real Power"/54(In54)
  [V29] -> " Real Power"/57(In57)
  [I26] -> " Real Power"/52(In52)
  [I28] -> " Real Power"/56(In56)
  [I26] -> " Reactive Power"/52(In52)
  [I25] -> " Real Power"/50(In50)
  [I20] -> " Reactive Power"/40(In40)
  [V19] -> " Reactive Power"/37(In37)
  " Reactive Power"/23(Out23) -> Reactive Power/23
  [I15] -> " Reactive Power"/30(In30)
  [V27] -> " Real Power"/53(In53)
  " Real Power"/19(Out19) -> Real Power/19
  " Reactive Power"/26(Out26) -> Reactive Power/26
  [V26] -> " Real Power"/51(In51)
  " Reactive Power"/13(Out13) -> Reactive Power/13
  [V20] -> " Real Power"/39(In39)
  [I24] -> " Real Power"/48(In48)
  [V25] -> " Real Power"/49(In49)
  " Reactive Power"/9(Out9) -> Reactive Power/9
  [V23] -> " Real Power"/45(In45)
  " Reactive Power"/25(Out25) -> Reactive Power/25
  [I8] -> " Real Power"/16(In16)
  [V30] -> " Real Power"/59(In59)
  [V16] -> " Real Power"/31(In31)
  [V1] -> " Reactive Power"/1(In1)
  [I17] -> " Real Power"/34(In34)
  [I28] -> " Reactive Power"/56(In56)
  [I22] -> " Real Power"/44(In44)
  [I23] -> " Real Power"/46(In46)
  [I23] -> " Reactive Power"/46(In46)
  " Reactive Power"/29(Out29) -> Reactive Power/29
  [I16] -> " Real Power"/32(In32)
  [V28] -> " Reactive Power"/55(In55)
  [V8] -> " Real Power"/15(In15)
  " Real Power"/22(Out22) -> Real Power/22
  [I30] -> " Reactive Power"/60(In60)
  " Real Power"/10(Out10) -> Real Power/10
  [V29] -> " Reactive Power"/57(In57)
  [V25] -> " Reactive Power"/49(In49)
  " Real Power"/7(Out7) -> Real Power/7
  " Real Power"/9(Out9) -> Real Power/9
  [V27] -> " Reactive Power"/53(In53)
  [V24] -> " Real Power"/47(In47)
  [I7] -> " Real Power"/14(In14)
  [V28] -> " Real Power"/55(In55)
  [I24] -> " Reactive Power"/48(In48)
  [I4] -> " Reactive Power"/8(In8)
  [I29] -> " Reactive Power"/58(In58)
  " Reactive Power"/22(Out22) -> Reactive Power/22
  [I25] -> " Reactive Power"/50(In50)
  [I13] -> " Reactive Power"/26(In26)
  " Reactive Power"/16(Out16) -> Reactive Power/16
  " Real Power"/8(Out8) -> Real Power/8
  " Reactive Power"/24(Out24) -> Reactive Power/24
  " Reactive Power"/28(Out28) -> Reactive Power/28
  " Real Power"/4(Out4) -> Real Power/4
  [I5] -> " Real Power"/10(In10)
  " Real Power"/20(Out20) -> Real Power/20
  [V19] -> " Real Power"/37(In37)
  [V8] -> " Reactive Power"/15(In15)
  " Reactive Power"/2(Out2) -> Reactive Power/2
  [V7] -> " Real Power"/13(In13)
  " Real Power"/18(Out18) -> Real Power/18
  connections:
  Gen1/RConn3 -- Three-Phase Transformer (Two Windings)/LConn3
  Gen1/RConn2 -- Three-Phase Transformer (Two Windings)/LConn2
  Gen1/RConn1 -- Three-Phase Transformer (Two Windings)/LConn1
  Gen3/RConn1 -- Three-Phase Transformer (Two Windings)2/LConn1
  Gen3/RConn2 -- Three-Phase Transformer (Two Windings)2/LConn2
  Gen3/RConn3 -- Three-Phase Transformer (Two Windings)2/LConn3
  Gen4/RConn1 -- Three-Phase Transformer (Two Windings)3/LConn1
  Gen4/RConn2 -- Three-Phase Transformer (Two Windings)3/LConn2
  Gen4/RConn3 -- Three-Phase Transformer (Two Windings)3/LConn3
  Gen5/RConn1 -- Three-Phase Transformer (Two Windings)4/LConn1
  Gen5/RConn2 -- Three-Phase Transformer (Two Windings)4/LConn2
  Gen5/RConn3 -- Three-Phase Transformer (Two Windings)4/LConn3
  Gen6/RConn1 -- Three-Phase Transformer (Two Windings)5/LConn1
  Gen6/RConn2 -- Three-Phase Transformer (Two Windings)5/LConn2
  Gen6/RConn3 -- Three-Phase Transformer (Two Windings)5/LConn3
  Three-Phase Series RLC Load1/LConn1 -- Bus 3/RConn1
  Three-Phase Series RLC Load1/LConn2 -- Bus 3/RConn2
  Three-Phase Series RLC Load1/LConn3 -- Bus 3/RConn3
  Three-Phase Series RLC Load2/LConn2 -- Bus 4/RConn2
  Three-Phase Series RLC Load2/LConn3 -- Bus 4/RConn3
  Three-Phase Series RLC Load2/LConn1 -- Bus 4/RConn1
  Three-Phase Series RLC Load5/LConn2 -- Bus 7/RConn2
  Three-Phase Series RLC Load5/LConn3 -- Bus 7/RConn3
  Three-Phase Series RLC Load5/LConn1 -- Bus 7/RConn1
  Three-Phase Series RLC Load7/LConn3 -- Bus 10/RConn3
  Three-Phase Series RLC Load7/LConn2 -- Bus 10/RConn2
  Three-Phase Series RLC Load7/LConn1 -- Bus 10/RConn1
  Three-Phase Series RLC Load9/LConn3 -- Bus 12/RConn3
  Three-Phase Series RLC Load9/LConn2 -- Bus 12/RConn2
  Three-Phase Series RLC Load9/LConn1 -- Bus 12/RConn1
  Three-Phase Series RLC Load10/LConn3 -- Bus 14/RConn3
  Three-Phase Series RLC Load10/LConn2 -- Bus 14/RConn2
  Three-Phase Series RLC Load10/LConn1 -- Bus 14/RConn1
  Three-Phase Series RLC Load11/LConn3 -- Bus 15/RConn3
  Three-Phase Series RLC Load11/LConn2 -- Bus 15/RConn2
  Three-Phase Series RLC Load11/LConn1 -- Bus 15/RConn1
  Three-Phase Transformer (Two Windings)/RConn1 -- Bus 1/RConn1
  Three-Phase Transformer (Two Windings)/RConn2 -- Bus 1/RConn2
  Three-Phase Transformer (Two Windings)/RConn3 -- Bus 1/RConn3
  Three-Phase Series RLC Load/LConn1 -- Bus 2/RConn1 -- Three-Phase Fault2/LConn1 -- Three-Phase Transformer (Two Windings)1/RConn1
  Three-Phase Series RLC Load/LConn3 -- Bus 2/RConn3 -- Three-Phase Series RLC Load/LConn2 -- Three-Phase Transformer (Two Windings)1/RConn2 -- Three-Phase Fault2/LConn2 -- Bus 2/RConn2 -- Three-Phase Fault2/LConn3 -- Three-Phase Transformer (Two Windings)1/RConn3
  Three-Phase Transformer (Two Windings)2/RConn1 -- Three-Phase Series RLC Load3/LConn1 -- Three-Phase Fault1/LConn1 -- Bus 5/RConn1
  Three-Phase Transformer (Two Windings)2/RConn2 -- Three-Phase Series RLC Load3/LConn2 -- Three-Phase Fault1/LConn2 -- Bus 5/RConn2
  Three-Phase Transformer (Two Windings)2/RConn3 -- Three-Phase Series RLC Load3/LConn3 -- Three-Phase Fault1/LConn3 -- Bus 5/RConn3
  Three-Phase Transformer (Two Windings)3/RConn1 -- Three-Phase Series RLC Load12/LConn1 -- Bus 8/RConn1
  Three-Phase Transformer (Two Windings)3/RConn2 -- Three-Phase Series RLC Load12/LConn2 -- Bus 8/RConn2
  Three-Phase Transformer (Two Windings)3/RConn3 -- Three-Phase Series RLC Load12/LConn3 -- Bus 8/RConn3
  Three-Phase Transformer (Two Windings)4/RConn1 -- Bus 11/RConn1
  Three-Phase Transformer (Two Windings)4/RConn2 -- Bus 11/RConn2
  Three-Phase Transformer (Two Windings)4/RConn3 -- Bus 11/RConn3
  Three-Phase Transformer (Two Windings)5/RConn1 -- Bus 13/RConn1
  Three-Phase Transformer (Two Windings)5/RConn2 -- Bus 13/RConn2
  Three-Phase Transformer (Two Windings)5/RConn3 -- Bus 13/RConn3
  Three-Phase Series RLC Branch/LConn1 -- Three-Phase Series RLC Branch1/LConn1 -- Bus 1/LConn1
  Three-Phase Series RLC Branch/LConn2 -- Three-Phase Series RLC Branch1/LConn2 -- Bus 1/LConn2
  Three-Phase Series RLC Branch/LConn3 -- Three-Phase Series RLC Branch1/LConn3 -- Bus 1/LConn3
  Three-Phase Series RLC Branch/RConn1 -- Three-Phase Series RLC Branch5/LConn1 -- Three-Phase Series RLC Branch4/LConn1 -- Three-Phase Series RLC Branch3/LConn1 -- Bus 2/LConn1
  Three-Phase Series RLC Branch/RConn2 -- Three-Phase Series RLC Branch5/LConn2 -- Three-Phase Series RLC Branch4/LConn2 -- Three-Phase Series RLC Branch3/LConn2 -- Bus 2/LConn2
  Three-Phase Series RLC Branch/RConn3 -- Three-Phase Series RLC Branch5/LConn3 -- Three-Phase Series RLC Branch4/LConn3 -- Three-Phase Series RLC Branch3/LConn3 -- Bus 2/LConn3
  Three-Phase Series RLC Branch1/RConn1 -- Three-Phase Series RLC Branch2/LConn1 -- Bus 3/LConn1
  Three-Phase Series RLC Branch1/RConn2 -- Three-Phase Series RLC Branch2/LConn2 -- Bus 3/LConn2
  Three-Phase Series RLC Branch1/RConn3 -- Three-Phase Series RLC Branch2/LConn3 -- Bus 3/LConn3
  Three-Phase Series RLC Branch2/RConn1 -- Three-Phase Series RLC Branch17/LConn1 -- Three-Phase Series RLC Branch3/RConn1 -- Three-Phase Series RLC Branch6/LConn1 -- Bus 4/LConn1
  Three-Phase Series RLC Branch2/RConn2 -- Three-Phase Series RLC Branch17/LConn2 -- Three-Phase Series RLC Branch3/RConn2 -- Three-Phase Series RLC Branch6/LConn2 -- Bus 4/LConn2
  Three-Phase Series RLC Branch2/RConn3 -- Three-Phase Series RLC Branch17/LConn3 -- Three-Phase Series RLC Branch3/RConn3 -- Three-Phase Series RLC Branch6/LConn3 -- Bus 4/LConn3
  Bus 5/LConn1 -- Three-Phase Series RLC Branch8/LConn1 -- Three-Phase Series RLC Branch4/RConn1
  Bus 5/LConn2 -- Three-Phase Series RLC Branch8/LConn2 -- Three-Phase Series RLC Branch4/RConn2
  Bus 5/LConn3 -- Three-Phase Series RLC Branch8/LConn3 -- Three-Phase Series RLC Branch4/RConn3
  Bus 6/LConn1 -- Three-Phase Series RLC Branch6/RConn1 -- Three-Phase Series RLC Branch9/LConn1 -- Three-Phase Series RLC Branch10/LConn1 -- Three-Phase Series RLC Branch5/RConn1 -- Three-Phase Series RLC Branch37/LConn1 -- Three-Phase Series RLC Branch12/LConn1
  Bus 6/LConn2 -- Three-Phase Series RLC Branch6/RConn2 -- Three-Phase Series RLC Branch9/LConn2 -- Three-Phase Series RLC Branch10/LConn2 -- Three-Phase Series RLC Branch12/LConn2 -- Three-Phase Series RLC Branch5/RConn2 -- Three-Phase Series RLC Branch37/LConn2
  Bus 6/LConn3 -- Three-Phase Series RLC Branch6/RConn3 -- Three-Phase Series RLC Branch9/LConn3 -- Three-Phase Series RLC Branch10/LConn3 -- Three-Phase Series RLC Branch12/LConn3 -- Three-Phase Series RLC Branch5/RConn3 -- Three-Phase Series RLC Branch37/LConn3
  Three-Phase Series RLC Branch7/RConn1 -- Bus 7/LConn1 -- Three-Phase Series RLC Branch8/RConn1
  Three-Phase Series RLC Branch7/RConn2 -- Three-Phase Series RLC Branch8/RConn2 -- Bus 7/LConn2
  Three-Phase Series RLC Branch7/RConn3 -- Three-Phase Series RLC Branch8/RConn3 -- Bus 7/LConn3
  Three-Phase Series RLC Branch9/RConn1 -- Three-Phase Series RLC Branch38/LConn1 -- Bus 8/LConn1
  Three-Phase Series RLC Branch9/RConn2 -- Bus 8/LConn2 -- Three-Phase Series RLC Branch38/LConn2
  Three-Phase Series RLC Branch9/RConn3 -- Three-Phase Series RLC Branch38/LConn3 -- Bus 8/LConn3
  Three-Phase Series RLC Branch10/RConn1 -- Three-Phase Series RLC Branch13/LConn1 -- Bus 9/LConn1
  Three-Phase Series RLC Branch10/RConn2 -- Three-Phase Series RLC Branch13/LConn2 -- Bus 9/LConn2
  Three-Phase Series RLC Branch10/RConn3 -- Three-Phase Series RLC Branch13/LConn3 -- Bus 9/LConn3
  Three-Phase Series RLC Branch11/LConn1 -- Bus 9/RConn1
  Three-Phase Series RLC Branch11/LConn2 -- Bus 9/RConn2
  Three-Phase Series RLC Branch11/LConn3 -- Bus 9/RConn3
  Three-Phase Series RLC Branch11/RConn1 -- Three-Phase Series RLC Branch12/RConn1 -- Three-Phase Series RLC Branch25/LConn1 -- Three-Phase Series RLC Branch27/RConn1 -- Three-Phase Series RLC Branch24/LConn1 -- Three-Phase Series RLC Branch20/LConn1 -- Bus 10/LConn1
  Three-Phase Series RLC Branch11/RConn2 -- Three-Phase Series RLC Branch12/RConn2 -- Three-Phase Series RLC Branch25/LConn2 -- Three-Phase Series RLC Branch27/RConn2 -- Three-Phase Series RLC Branch24/LConn2 -- Three-Phase Series RLC Branch20/LConn2 -- Bus 10/LConn2
  Three-Phase Series RLC Branch11/RConn3 -- Three-Phase Series RLC Branch12/RConn3 -- Three-Phase Series RLC Branch25/LConn3 -- Three-Phase Series RLC Branch27/RConn3 -- Three-Phase Series RLC Branch24/LConn3 -- Three-Phase Series RLC Branch20/LConn3 -- Bus 10/LConn3
  Three-Phase Series RLC Branch13/RConn1 -- Bus 11/LConn1
  Three-Phase Series RLC Branch13/RConn2 -- Bus 11/LConn2
  Three-Phase Series RLC Branch13/RConn3 -- Bus 11/LConn3
  Three-Phase Series RLC Branch14/LConn1 -- Three-Phase Series RLC Branch39/LConn1 -- Three-Phase Series RLC Branch18/LConn1 -- Three-Phase Series RLC Branch15/LConn1 -- Bus 12/LConn1
  Three-Phase Series RLC Branch14/LConn2 -- Three-Phase Series RLC Branch39/LConn2 -- Three-Phase Series RLC Branch18/LConn2 -- Three-Phase Series RLC Branch15/LConn2 -- Bus 12/LConn2
  Three-Phase Series RLC Branch14/LConn3 -- Three-Phase Series RLC Branch39/LConn3 -- Three-Phase Series RLC Branch18/LConn3 -- Three-Phase Series RLC Branch15/LConn3 -- Bus 12/LConn3
  Three-Phase Series RLC Branch14/RConn1 -- Bus 13/LConn1
  Three-Phase Series RLC Branch14/RConn2 -- Bus 13/LConn2
  Three-Phase Series RLC Branch14/RConn3 -- Bus 13/LConn3
  Three-Phase Series RLC Branch15/RConn1 -- Three-Phase Series RLC Branch16/LConn1 -- Bus 14/LConn1
  Three-Phase Series RLC Branch15/RConn2 -- Three-Phase Series RLC Branch16/LConn2 -- Bus 14/LConn2
  Three-Phase Series RLC Branch15/RConn3 -- Three-Phase Series RLC Branch16/LConn3 -- Bus 14/LConn3
  Three-Phase Series RLC Branch16/RConn1 -- Three-Phase Series RLC Branch39/RConn1 -- Three-Phase Series RLC Branch21/LConn1 -- Three-Phase Series RLC Branch28/LConn1 -- Three-Phase Series RLC Branch17/RConn1 -- Bus 15/LConn1
  Three-Phase Series RLC Branch16/RConn2 -- Three-Phase Series RLC Branch39/RConn2 -- Three-Phase Series RLC Branch21/LConn2 -- Three-Phase Series RLC Branch28/LConn2 -- Three-Phase Series RLC Branch17/RConn2 -- Bus 15/LConn2
  Three-Phase Series RLC Branch16/RConn3 -- Three-Phase Series RLC Branch39/RConn3 -- Three-Phase Series RLC Branch21/LConn3 -- Three-Phase Series RLC Branch28/LConn3 -- Three-Phase Series RLC Branch17/RConn3 -- Bus 15/LConn3
  Three-Phase Series RLC Load8/LConn1 -- Bus 17/LConn1
  Three-Phase Series RLC Load8/LConn2 -- Bus 17/LConn2
  Three-Phase Series RLC Load8/LConn3 -- Bus 17/LConn3
  Three-Phase Series RLC Load13/LConn1 -- Bus 18/LConn1
  Three-Phase Series RLC Load13/LConn2 -- Bus 18/LConn2
  Three-Phase Series RLC Load13/LConn3 -- Bus 18/LConn3
  Three-Phase Series RLC Load14/LConn1 -- Bus 19/LConn1
  Three-Phase Series RLC Load14/LConn2 -- Bus 19/LConn2
  Three-Phase Series RLC Load14/LConn3 -- Bus 19/LConn3
  Three-Phase Series RLC Load15/LConn1 -- Bus 20/LConn1
  Three-Phase Series RLC Load15/LConn2 -- Bus 20/LConn2
  Three-Phase Series RLC Load15/LConn3 -- Bus 20/LConn3
  Three-Phase Series RLC Load17/LConn1 -- Bus 23/LConn1
  Three-Phase Series RLC Load17/LConn2 -- Bus 23/LConn2
  Three-Phase Series RLC Load17/LConn3 -- Bus 23/LConn3
  Three-Phase Series RLC Load18/LConn1 -- Bus 24/LConn1
  Three-Phase Series RLC Load18/LConn2 -- Bus 24/LConn2
  Three-Phase Series RLC Load18/LConn3 -- Bus 24/LConn3
  Three-Phase Series RLC Load19/LConn1 -- Bus 26/LConn1
  Three-Phase Series RLC Load19/LConn2 -- Bus 26/LConn2
  Three-Phase Series RLC Load19/LConn3 -- Bus 26/LConn3
  Three-Phase Series RLC Load21/LConn1 -- Bus 29/LConn1
  Three-Phase Series RLC Load21/LConn2 -- Bus 29/LConn2
  Three-Phase Series RLC Load21/LConn3 -- Bus 29/LConn3
  Three-Phase Series RLC Load22/LConn1 -- Bus 30/LConn1
  Three-Phase Series RLC Load22/LConn2 -- Bus 30/LConn2
  Three-Phase Series RLC Load22/LConn3 -- Bus 30/LConn3
  Three-Phase Series RLC Branch18/RConn1 -- Three-Phase Series RLC Branch19/LConn1 -- Three-Phase Series RLC Branch19/LConn2 -- Three-Phase Series RLC Branch19/LConn3 -- Bus 16/RConn1
  Three-Phase Series RLC Branch18/RConn2 -- Bus 16/RConn2
  Three-Phase Series RLC Branch18/RConn3 -- Bus 16/RConn3
  Three-Phase Series RLC Branch19/RConn1 -- Three-Phase Series RLC Branch20/RConn1 -- Bus 17/RConn1
  Three-Phase Series RLC Branch19/RConn2 -- Three-Phase Series RLC Branch20/RConn2 -- Bus 17/RConn2
  Three-Phase Series RLC Branch19/RConn3 -- Three-Phase Series RLC Branch20/RConn3 -- Bus 17/RConn3
  Three-Phase Series RLC Branch21/RConn1 -- Bus 18/RConn1 -- Three-Phase Series RLC Branch22/LConn1
  Three-Phase Series RLC Branch21/RConn2 -- Bus 18/RConn2 -- Three-Phase Series RLC Branch22/LConn2
  Three-Phase Series RLC Branch21/RConn3 -- Bus 18/RConn3 -- Three-Phase Series RLC Branch22/LConn3
  Three-Phase Series RLC Branch22/RConn1 -- Bus 19/RConn1 -- Three-Phase Series RLC Branch23/LConn1
  Three-Phase Series RLC Branch22/RConn2 -- Bus 19/RConn2 -- Three-Phase Series RLC Branch23/LConn2
  Three-Phase Series RLC Branch22/RConn3 -- Bus 19/RConn3 -- Three-Phase Series RLC Branch23/LConn3
  Three-Phase Series RLC Branch23/RConn1 -- Bus 20/RConn1 -- Three-Phase Series RLC Branch24/RConn1
  Three-Phase Series RLC Branch23/RConn2 -- Bus 20/RConn2 -- Three-Phase Series RLC Branch24/RConn2
  Three-Phase Series RLC Branch23/RConn3 -- Bus 20/RConn3 -- Three-Phase Series RLC Branch24/RConn3
  Three-Phase Series RLC Load16/LConn3 -- Bus 21/LConn3
  Three-Phase Series RLC Load16/LConn2 -- Bus 21/LConn2
  Three-Phase Series RLC Load16/LConn1 -- Bus 21/LConn1
  Three-Phase Series RLC Branch25/RConn1 -- Bus 21/RConn1 -- Three-Phase Series RLC Branch26/LConn1
  Three-Phase Series RLC Branch25/RConn2 -- Bus 21/RConn2 -- Three-Phase Series RLC Branch26/LConn2
  Three-Phase Series RLC Branch25/RConn3 -- Bus 21/RConn3 -- Three-Phase Series RLC Branch26/LConn3
  Three-Phase Series RLC Branch26/RConn1 -- Bus 22/RConn1 -- Three-Phase Series RLC Branch29/LConn1
  Three-Phase Series RLC Branch26/RConn2 -- Bus 22/RConn2 -- Three-Phase Series RLC Branch29/LConn2
  Three-Phase Series RLC Branch26/RConn3 -- Bus 22/RConn3 -- Three-Phase Series RLC Branch29/LConn3
  Three-Phase Series RLC Branch28/RConn1 -- Three-Phase Series RLC Branch30/LConn1 -- Bus 23/RConn1
  Three-Phase Series RLC Branch28/RConn2 -- Three-Phase Series RLC Branch30/LConn2 -- Bus 23/RConn2
  Three-Phase Series RLC Branch28/RConn3 -- Three-Phase Series RLC Branch30/LConn3 -- Bus 23/RConn3
  Three-Phase Series RLC Branch29/RConn1 -- Three-Phase Series RLC Branch31/LConn1 -- Three-Phase Series RLC Branch30/RConn1 -- Bus 24/RConn1
  Three-Phase Series RLC Branch29/RConn2 -- Three-Phase Series RLC Branch31/LConn2 -- Three-Phase Series RLC Branch30/RConn2 -- Bus 24/RConn2
  Three-Phase Series RLC Branch29/RConn3 -- Three-Phase Series RLC Branch31/LConn3 -- Three-Phase Series RLC Branch30/RConn3 -- Bus 24/RConn3
  Three-Phase Series RLC Branch31/RConn1 -- Bus 25/RConn1
  Three-Phase Series RLC Branch31/RConn2 -- Bus 25/RConn2
  Three-Phase Series RLC Branch31/RConn3 -- Bus 25/RConn3
  Three-Phase Series RLC Branch32/LConn1 -- Three-Phase Series RLC Branch33/LConn1 -- Bus 25/LConn1
  Bus 25/LConn2 -- Three-Phase Series RLC Branch32/LConn2 -- Three-Phase Series RLC Branch33/LConn2
  Three-Phase Series RLC Branch32/LConn3 -- Three-Phase Series RLC Branch33/LConn3 -- Bus 25/LConn3
  Three-Phase Series RLC Branch32/RConn1 -- Bus 26/RConn1
  Three-Phase Series RLC Branch32/RConn2 -- Bus 26/RConn2
  Three-Phase Series RLC Branch32/RConn3 -- Bus 26/RConn3
  Three-Phase Series RLC Branch35/LConn1 -- Three-Phase Series RLC Branch34/LConn1 -- Three-Phase Series RLC Branch36/RConn1 -- Bus 27/RConn1
  Three-Phase Series RLC Branch35/LConn2 -- Three-Phase Series RLC Branch34/LConn2 -- Three-Phase Series RLC Branch36/RConn2 -- Bus 27/RConn2
  Three-Phase Series RLC Branch35/LConn3 -- Three-Phase Series RLC Branch34/LConn3 -- Three-Phase Series RLC Branch36/RConn3 -- Bus 27/RConn3
  Three-Phase Series RLC Branch34/RConn1 -- Three-Phase Series RLC Branch40/LConn1 -- Bus 29/RConn1
  Three-Phase Series RLC Branch34/RConn2 -- Three-Phase Series RLC Branch40/LConn2 -- Bus 29/RConn2
  Three-Phase Series RLC Branch34/RConn3 -- Three-Phase Series RLC Branch40/LConn3 -- Bus 29/RConn3
  Three-Phase Series RLC Branch35/RConn1 -- Three-Phase Series RLC Branch40/RConn1 -- Bus 30/RConn1
  Three-Phase Series RLC Branch35/RConn2 -- Three-Phase Series RLC Branch40/RConn2 -- Bus 30/RConn2
  Three-Phase Series RLC Branch35/RConn3 -- Three-Phase Series RLC Branch40/RConn3 -- Bus 30/RConn3
  Bus 28/LConn1 -- Three-Phase Series RLC Branch36/LConn1
  Bus 28/LConn2 -- Three-Phase Series RLC Branch36/LConn2
  Bus 28/LConn3 -- Three-Phase Series RLC Branch36/LConn3
  Bus 28/RConn1 -- Three-Phase Series RLC Branch38/RConn1 -- Three-Phase Series RLC Branch37/RConn1
  Bus 28/RConn2 -- Three-Phase Series RLC Branch38/RConn2 -- Three-Phase Series RLC Branch37/RConn2
  Bus 28/RConn3 -- Three-Phase Series RLC Branch38/RConn3 -- Three-Phase Series RLC Branch37/RConn3
  Three-Phase Series RLC Branch27/LConn2 -- Bus 22/LConn2
  Bus 22/LConn3 -- Three-Phase Series RLC Branch27/LConn3
  Bus 22/LConn1 -- Three-Phase Series RLC Branch27/LConn1
  Three-Phase Series RLC Branch7/LConn1 -- Bus 6/RConn1
  Three-Phase Series RLC Branch7/LConn2 -- Bus 6/RConn2
  Three-Phase Series RLC Branch7/LConn3 -- Bus 6/RConn3
  Three-Phase Series RLC Branch33/RConn1 -- Bus 27/LConn1
  Three-Phase Series RLC Branch33/RConn2 -- Bus 27/LConn2
  Three-Phase Series RLC Branch33/RConn3 -- Bus 27/LConn3
  Three-Phase Transformer (Two Windings)1/LConn3 -- Gen2/RConn3
  Gen2/RConn2 -- Three-Phase Transformer (Two Windings)1/LConn2
  Three-Phase Transformer (Two Windings)1/LConn1 -- Gen2/RConn1
  Bus 16/LConn1 -- Three-Phase Series RLC Load4/LConn1
  Bus 16/LConn2 -- Three-Phase Series RLC Load4/LConn2
  Bus 16/LConn3 -- Three-Phase Series RLC Load4/LConn3
